simulink model "uniciclo_FL2"  (R2020a)
settings: Solver=VariableStepAuto  StartTime=0.0  StopTime=Inf  MaxStep=0.01  RelTol=1e-3
InitFcn:
  | init_uniciclo
StopFcn:
  | stop_uniciclo
values from neighbouring files (symbols this model uses):
  K1 = [100; 100]    [init_uniciclo.m]
  K2 = [100; 100]    [init_uniciclo.m]
  theta_iniziale = pi/3    (= 1.0471975512)    [init_uniciclo.m]
  v = out.state_ts.Data(:,4)    [stop_uniciclo.m]
  v_iniziale = 1    [init_uniciclo.m]
  x_p_finale = 0    [init_uniciclo.m]
  x_p_iniziale = 10    [init_uniciclo.m]
  y_p_finale = 0    [init_uniciclo.m]
  y_p_iniziale = -20    [init_uniciclo.m]
undefined symbols (not defined in the file or in its folder): a, indexclot, Lsofar, Lsofarclot, n_p, s_f, t_f, theta_rette, v_raggiunta, xp, yp
libraries: simulink x1
settings Model: Creator=Andrea_Ferroni  LastModifiedBy=9ales

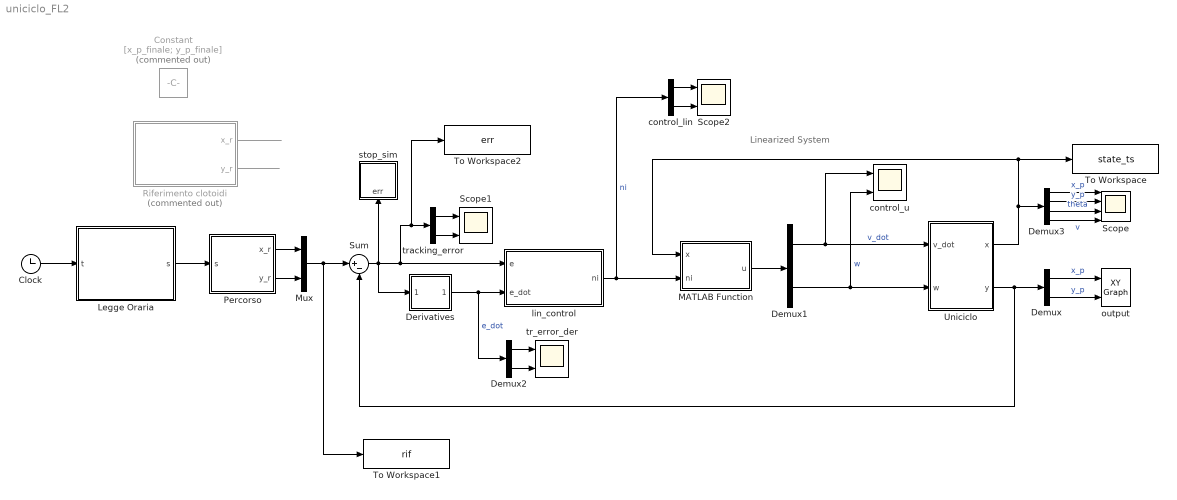
== system uniciclo_FL2 ==
  note: Linearized System
  Clock : Clock
  Constant : Constant  Commented=on  Value=[x_p_finale; y_p_finale]
  Demux : Demux  Outputs=2
  Demux1 : Demux  Outputs=2
  Demux2 : Demux  Outputs=2
  Demux3 : Demux
  Derivatives : Subsystem
  Legge Oraria : MATLAB Function  TreatAsAtomicUnit=on
  MATLAB Function : MATLAB Function  TreatAsAtomicUnit=on
  Mux : Mux  Inputs=2
  Percorso : MATLAB Function  TreatAsAtomicUnit=on
  Riferimento clotoidi : Subsystem  Commented=on
  Scope : Scope  NumInputPorts=4
  Scope1 : Scope  NumInputPorts=2
  Scope2 : Scope  NumInputPorts=2
  Sum : Sum  Inputs=|+-
  To Workspace : ToWorkspace  VariableName=state_ts  SaveFormat=Timeseries  SampleTime=-1
  To Workspace1 : ToWorkspace  VariableName=rif  SaveFormat=Timeseries  SampleTime=-1
  To Workspace2 : ToWorkspace  VariableName=err  SaveFormat=Timeseries  SampleTime=-1
  Uniciclo : Subsystem
      mask Display: image('$imagefile'); % Use "Edit Image" on toolstrip to change.
  control_lin : Demux  Outputs=2
  control_u : Scope  NumInputPorts=2
  lin_control : MATLAB Function  TreatAsAtomicUnit=on
  output : simulink/Sinks/XY Graph  xmin=-50  xmax=50  ymin=-50  ymax=50  st=-1
  stop_sim : Subsystem
  tr_error_der : Scope  NumInputPorts=2
  tracking_error : Demux  Outputs=2
  wires:
  Uniciclo/1(x) -> Demux3/1, To Workspace/1, MATLAB Function/1(x)
  Mux/1 -> Sum/1, To Workspace1/1
  Uniciclo/2(y) -> Demux/1, Sum/2
  lin_control/1(ni) -> control_lin/1, MATLAB Function/2(ni)  "ni"
  Sum/1 -> Derivatives/1(In1), lin_control/1(e), To Workspace2/1, tracking_error/1, stop_sim/1(err)
  Derivatives/1(Out1) -> Demux2/1, lin_control/2(e_dot)  "e_dot"
  Demux/1 -> output/1  "x_p"
  Demux/2 -> output/2  "y_p"
  Demux2/1 -> tr_error_der/1
  Demux2/2 -> tr_error_der/2
  tracking_error/1 -> Scope1/1
  tracking_error/2 -> Scope1/2
  MATLAB Function/1(u) -> Demux1/1
  Demux1/1 -> control_u/1, Uniciclo/1(v_dot)  "v_dot"
  Demux1/2 -> control_u/2, Uniciclo/2(w)  "w"
  control_lin/2 -> Scope2/2
  control_lin/1 -> Scope2/1
  Demux3/1 -> Scope/1  "x_p"
  Demux3/2 -> Scope/2  "y_p"
  Demux3/3 -> Scope/3  "theta"
  Demux3/4 -> Scope/4  "v"
  Riferimento clotoidi/1(x_r) -> ?
  Riferimento clotoidi/2(y_r) -> ?
  Clock/1 -> Legge Oraria/1(t)
  Legge Oraria/1(s) -> Percorso/1(s)
  Percorso/1(x_r) -> Mux/1
  Percorso/2(y_r) -> Mux/2

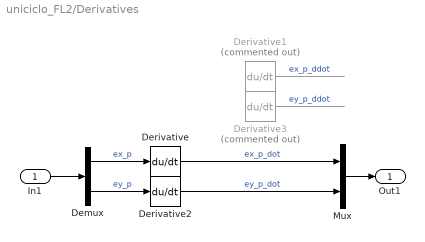
== system uniciclo_FL2/Derivatives ==
  In1 : Inport
  Demux : Demux  Outputs=2
  Derivative : Derivative  CoefficientInTFapproximation=1e10
  Derivative1 : Derivative  Commented=on  CoefficientInTFapproximation=1e10
  Derivative2 : Derivative  CoefficientInTFapproximation=1e10
  Derivative3 : Derivative  Commented=on  CoefficientInTFapproximation=1e10
  Mux : Mux  Inputs=2
  Out1 : Outport
  wires:
  In1/1 -> Demux/1
  Demux/1 -> Derivative/1  "ex_p"
  Derivative/1 -> Mux/1  "ex_p_dot"
  Derivative2/1 -> Mux/2  "ey_p_dot"
  Demux/2 -> Derivative2/1  "ey_p"
  Derivative1/1 -> ?  "ex_p_ddot"
  Derivative3/1 -> ?  "ey_p_ddot"
  Mux/1 -> Out1/1

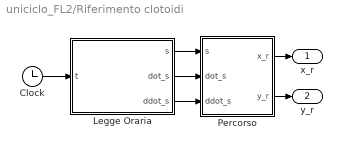
== system uniciclo_FL2/Riferimento clotoidi ==
  Clock : Clock
  Legge Oraria : MATLAB Function  TreatAsAtomicUnit=on
  Percorso : MATLAB Function  TreatAsAtomicUnit=on
  x_r : Outport
  y_r : Outport  Port=2
  wires:
  Clock/1 -> Legge Oraria/1(t)
  Legge Oraria/2(dot_s) -> Percorso/2(dot_s)
  Legge Oraria/1(s) -> Percorso/1(s)
  Legge Oraria/3(ddot_s) -> Percorso/3(ddot_s)
  Percorso/1(x_r) -> x_r/1
  Percorso/2(y_r) -> y_r/1

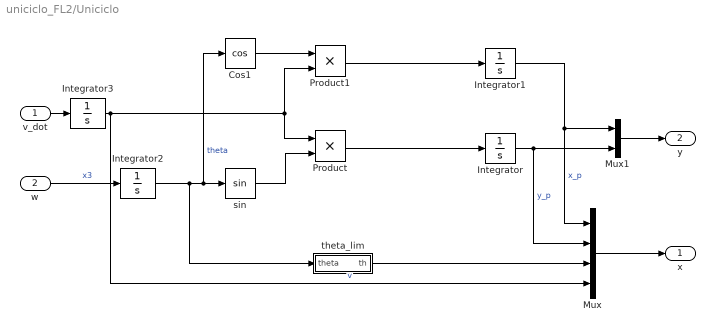
== system uniciclo_FL2/Uniciclo ==
  v_dot : Inport
  w : Inport  Port=2
  Cos1 : Trigonometry  Operator=cos
  Integrator : Integrator  InitialCondition=y_p_iniziale
  Integrator1 : Integrator  InitialCondition=x_p_iniziale
  Integrator2 : Integrator  InitialCondition=theta_iniziale
  Integrator3 : Integrator  InitialCondition=v_iniziale
  Mux : Mux
  Mux1 : Mux  Inputs=2
  Product : Product
  Product1 : Product
  sin : Trigonometry
  theta_lim : MATLAB Function  TreatAsAtomicUnit=on
  x : Outport
  y : Outport  Port=2
  wires:
  v_dot/1 -> Integrator3/1
  Cos1/1 -> Product1/1
  Product1/1 -> Integrator1/1
  Product/1 -> Integrator/1
  w/1 -> Integrator2/1  "x3"
  Integrator2/1 -> theta_lim/1(theta), Cos1/1, sin/1  "theta"
  sin/1 -> Product/2
  Mux/1 -> x/1
  Integrator1/1 -> Mux/1, Mux1/1  "x_p"
  Integrator/1 -> Mux/2, Mux1/2  "y_p"
  Mux1/1 -> y/1
  Integrator3/1 -> Mux/4, Product1/2, Product/1  "v"
  theta_lim/1(th) -> Mux/3

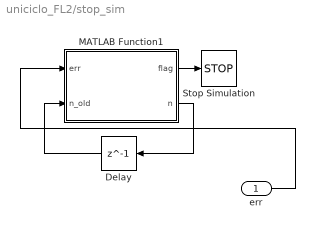
== system uniciclo_FL2/stop_sim ==
  err : Inport
  Delay : Delay  DelayLength=1
  MATLAB Function1 : MATLAB Function  TreatAsAtomicUnit=on
  Stop Simulation : Stop
  wires:
  MATLAB Function1/2(n) -> Delay/1
  MATLAB Function1/1(flag) -> Stop Simulation/1
  err/1 -> MATLAB Function1/1(err)
  Delay/1 -> MATLAB Function1/2(n_old)

== matlab function uniciclo_FL2/lin_control ==
  data: e input; ni output; e_dot input; K1 parameter size=[2,1]; K2 parameter size=[2,1]
function ni = lin_control(e, e_dot, K1, K2)

ni = K1.*e + K2.*e_dot;

end

== matlab function uniciclo_FL2/MATLAB Function ==
  data: x input; ni input; u output
function u = Linearized(x,ni)
theta = x(3);
v = x(4);

E_inv = inv_E(theta, v);
G = Gamma();
u =  -E_inv*G + E_inv*ni;
end

% gamma
function Gm = Gamma()
Gm = [0;0];
end
% 
function E_in = inv_E(theta, v)
E = [cos(theta) -v*sin(theta);
	 sin(theta)  v*cos(theta)];
E_in = inv(E);
end

== matlab function uniciclo_FL2/Riferimento clotoidi/Legge Oraria ==
  data: t input; s output; dot_s output; ddot_s output; v_iniziale parameter
function [s, dot_s, ddot_s] = legge_oraria(t,v_iniziale)
%#codegen PEPO

s = v_iniziale*t;
dot_s = v_iniziale;
ddot_s = 0.0;

%     if v_raggiunta==0
%         
%         if t<=(s_f/a)^0.5               %acce
%             s= 0.5*a*t^2;
%             dot_s=a*t;
%             ddot_s=a;
%             
%         elseif t>(s_f/a)^0.5 & t<=t_f   %decel
%             s=s_f-0.5*a*(t_f-t)^2;
%             dot_s=-a*t;
%             ddot_s=-a;
%             
%         end
%     
%     else    
%         
%         if t<=v/a                       %acc
%             s=0.5*a*t^2;
%             dot_s=a*t;
%             ddot_s=a;
%             
%         elseif t>v/a & t<=t_f-v/a       %v=cost
%             s=0.5*a*(v/a)^2 + v *(t-v/a);
%             dot_s=v;
%             ddot_s=0;
%             
%         elseif t>t_f-v/a & t<=t_f       %decel
%             s=s_f-0.5*a*(t_f-t)^2;
%             dot_s=v-a*(t - (t_f-v/a));
%             ddot_s=-a;
%             
%             
%         end
%             
%     end

end

== matlab function uniciclo_FL2/Uniciclo/theta_lim ==
  data: theta input; th output
function th = theta_lim(theta)
c = cos(theta);
s = sin(theta);
th = atan2(s, c);

== matlab function uniciclo_FL2/stop_sim/MATLAB Function1 ==
  data: flag output; err input; n output; n_old input; threshold parameter
function [flag, n] = stop_function(err, n_old, threshold)
	flag = 0;
	n = n_old;
	if norm(err, 2) < threshold
		n=n+1;
	else
		n=0;
	end
	
	if n > 10
		flag = 1;
		n = 0;
	end
end

== matlab function uniciclo_FL2/Riferimento clotoidi/Percorso ==
  data: s input; x_r output; dot_s input; ddot_s input; y_r output; a parameter; indexclot parameter; Lsofar parameter; Lsofarclot parameter; n_p parameter; s_f parameter; t_f parameter; theta_rette parameter; v parameter; v_raggiunta parameter; xp parameter; yp parameter
function [x_r,y_r ] = percorso(s, dot_s,ddot_s, a, indexclot, Lsofar, Lsofarclot, n_p, s_f, t_f, theta_rette, v, v_raggiunta, xp, yp)
%#codegen      PEPO


coder.extrinsic('pointsOnClothoid')

% v_r = dot_s ;
ntratto=0;
XYS=[0 0]'; %definito prima
%clot=struct('x0', 0, 'y0', 0, 'theta0', 0 , 'k0', 0, 'dk', 0, 'L', 0 );

%Parte per capire in che tratto sono
    if s<Lsofar(1)
        ntratto=1;
    else
    	for ii=2:(n_p-1)
        	if s>=Lsofar(ii-1) && s<=Lsofar(ii)
                ntratto=ii;
            end
    	end
    end

    
    
%calcolo delle coordinate x e y riferite a s e a ntratto
    if mod(ntratto,2)==1            %tratti dispari
        if ntratto==1
            XYS=[xp(ntratto)+cos(theta_rette(ntratto))*(s), yp(ntratto)+sin(theta_rette(ntratto))*(s)]';
        else
            XYS=[xp(ntratto)+cos(theta_rette(ntratto))*(s-Lsofar(ntratto-1)), yp(ntratto)+sin(theta_rette(ntratto))*(s-Lsofar(ntratto-1))]';
        end 

    elseif mod(ntratto,2)==0
        srel=s-Lsofar(ntratto-1);
        
        
        if srel<=Lsofarclot(ntratto/2).Lclot(1)
            XYS = double(pointsOnClothoid( indexclot(ntratto/2).clot.S0, srel ));
            
        elseif srel>Lsofarclot(ntratto/2).Lclot(1) & srel<=Lsofarclot(ntratto/2).Lclot(2)
            XYS = double(pointsOnClothoid( indexclot(ntratto/2).clot.SM, srel- indexclot(ntratto/2).clot.S0.L ));
            
        elseif srel>Lsofarclot(ntratto/2).Lclot(2)
            XYS = double(pointsOnClothoid( indexclot(ntratto/2).clot.S1, srel- indexclot(ntratto/2).clot.S0.L - indexclot(ntratto/2).clot.SM.L ));
        end
        
        
        
        %XYS = double(pointsOnClothoid( indexclot(ntratto/2).clot, s-Lsofar(ntratto-1) ));
        
    end

    x_r=XYS(1);
    y_r=XYS(2);

end

== matlab function uniciclo_FL2/Legge Oraria ==
  data: t input; s output; v_iniziale parameter
function s  = legge_oraria(t, v_iniziale)
%#codegen PEPO

s = v_iniziale*t;
dot_s = v_iniziale;
ddot_s = 0.0;

%     if v_raggiunta==0
%         
%         if t<=(s_f/a)^0.5               %acce
%             s= 0.5*a*t^2;
%             dot_s=a*t;
%             ddot_s=a;
%             
%         elseif t>(s_f/a)^0.5 & t<=t_f   %decel
%             s=s_f-0.5*a*(t_f-t)^2;
%             dot_s=-a*t;
%             ddot_s=-a;
%             
%         end
%     
%     else    
%         
%         if t<=v/a                       %acc
%             s=0.5*a*t^2;
%             dot_s=a*t;
%             ddot_s=a;
%             
%         elseif t>v/a & t<=t_f-v/a       %v=cost
%             s=0.5*a*(v/a)^2 + v *(t-v/a);
%             dot_s=v;
%             ddot_s=0;
%             
%         elseif t>t_f-v/a & t<=t_f       %decel
%             s=s_f-0.5*a*(t_f-t)^2;
%             dot_s=v-a*(t - (t_f-v/a));
%             ddot_s=-a;
%             
%             
%         end
%             
%     end

end

== matlab function uniciclo_FL2/Percorso ==
  data: s input; x_r output; y_r output
function [x_r, y_r] = percorso(s)

pos = s * [0; 1] + [1; 0]*cos(s); % sinusoide
% pos = [2;0]*cos(s) + [0;2]*sin(s); % circonferenza

x_r = pos(1);
y_r = pos(2);
end
